simulink model "ProcessNetworkSimulation"  (R2015b)
settings: Solver=VariableStepAuto  StartTime=0.0  StopTime=1000.0  RelTol=1e-3
libraries: simulink x1, simeventslib x1
(part 21 of 21)

== system ProcessNetworkSimulation/Process_99/Process ==
  OUTQueue : FIFOQueue  Capacity=inf
  ProcessQueue : FIFOQueue  Capacity=Inf  StatAverageWait=on  StatAverageQueueLength=on
      settings: OutputPortMap=o2,o3
  ProcessServer : NServer  NumberOfServers=16  ServiceTimeFrom=Signal port t  StatNumberDeparted=on  StatUtilization=on
      settings: OutputPortMap=o0,o5
  ProcessTime : EventBasedRandomNumber  meanExp=0.05  minUnif=1  meanNorm=2  stdNorm=0.2  Seed=39745
  Routing : EventBasedRandomNumber  Distribution=Arbitrary discrete  valueVecDisc=[0,1,2,3,4,5,6,7,8,9,10,11,12,13,14,15,16,17,18,19,20,21,22,23,24,25,26,27,28,29,30,31,32,33,34,35,36,37,38,39,40]  probVecDisc=[0,0.0369,0.0082,0.0369,0.0369,0.0369,0.0082,0.0406,0.0287,0.0328,0.0369,0.0205,0.0287,0.0369,0.0287,0.0123,0.0287,0.0369,0.0287,0.0082,0.0246,0.0205,0.041,0.0082,0.0082,0.0205,0.0287,0.0246,0.0123,0.0082,0.0369,0.0082,0.0123,0.0287,0.041,0.0246,0.041,0.0205,0.0287,0.0287,0]  Seed=42962
  read_ProcessTimer : ReadTimer  TimerTag=T_Process_99  StatAverageTimeElapsed=on
      settings: OutputPortMap=o3
  setRouting : SetAttribute  AttributeName=outputFlowNode  AttributeFrom=Signal port  EvaluatedAttributeValue={ []}
  start_ProcessTimer : StartTimer  TimerTag=T_Process_99  TimerStartedOption=Restart
  IN_Job : PMIOPort  Port=1  Side=Left
  OUT_Job : PMIOPort  Port=2  Side=Right
  wires:
  Routing/1 -> setRouting/1
  ProcessTime/1 -> ProcessServer/1
  connections:
  setRouting/LConn1 -- OUTQueue/RConn1
  IN_Job/RConn1 -- start_ProcessTimer/LConn1
  ProcessServer/RConn1 -- read_ProcessTimer/LConn1
  start_ProcessTimer/RConn1 -- ProcessQueue/LConn1
  ProcessQueue/RConn1 -- ProcessServer/LConn1
  read_ProcessTimer/RConn1 -- OUTQueue/LConn1
  OUT_Job/RConn1 -- setRouting/RConn1
